simulink library "simCryogenics_lib"  (R2016a)
settings: Solver=VariableStepAuto  StartTime=0.0  StopTime=10.0  RelTol=1e-3
undefined symbols (not defined in the file or in its folder): gcbh, simscape
(part 4 of 4)

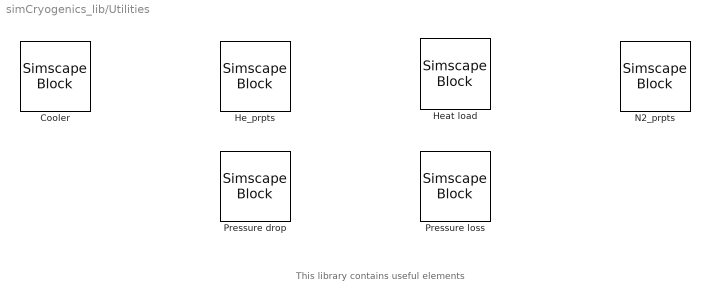
== system simCryogenics_lib/Utilities ==
  note: This library contains useful elements
  Cooler : SimscapeBlock  DialogController=NetworkEngine.DynNeDlgSource  LoadFcn=simscape.compiler.sli.internal.callback('LoadFcn',gcbh);  SourceFile=simCryogenics.Utilities.Cooler  mask(Cooler){ComponentPath=simCryogenics.Utilities.Cooler, ComponentVariants=simCryogenics.Utilities.Cooler, ComponentVariantNames=Cooler, ClassName=Cooler, SchemaVersion=1, Tout=300, Tout_unit=K, Tout_conf=compiletime}
      mask prompts: Tout "output temperature"
      mask help: This block is a cooler
      mask init:
      | simscape.compiler.sli.internal.preinitmask(gcb);
      settings: CopyFcn=simscape.compiler.sli.internal.callback('CopyFcn',gcbh);  DeleteFcn=simscape.compiler.sli.internal.callback('DeleteFcn',gcbh);  ModelCloseFcn=simscape.compiler.sli.internal.callback('ModelCloseFcn',gcbh);  PreSaveFcn=simscape.compiler.sli.internal.callback('PreSaveFcn',gcbh);  PostSaveFcn=simscape.compiler.sli.internal.callback('PostSaveFcn',gcbh);  PreCopyFcn=simscape.compiler.sli.internal.callback('PreCopyFcn',gcbh);  PreDeleteFcn=simscape.compiler.sli.internal.callback('PreDeleteFcn',gcbh);
      mask Help: web(nesl_help(gcbh))
      mask TypeOptions Tout_conf: compiletime | runtime
      mask Display:
      | disp('Simscape\n\n\n')
      | disp('\n\n\nCooler');
      | color('red');
      | port_label('RConn', 1,'out');
      | port_label('LConn', 1,'in');
  He_prpts : SimscapeBlock  DialogController=NetworkEngine.DynNeDlgSource  LoadFcn=simscape.compiler.sli.internal.callback('LoadFcn',gcbh);  SourceFile=simCryogenics.Utilities.He_prpts  mask(He_prpts){ComponentPath=simCryogenics.Utilities.He_prpts, ComponentVariants=simCryogenics.Utilities.He_prpts, ComponentVariantNames=He_prpts, ClassName=He_prpts, SchemaVersion=1, P_min=0.01, P_min_unit=bar, P_min_conf=compiletime, P_max=50, P_max_unit=bar, P_max_conf=compiletime, T_min=1, T_min_unit=K, T_min_conf=compiletime, T_max=100, T_max_unit=K, T_max_conf=compiletime, N=100, N_unit=1, N_conf=compiletime, Mol=4.0026 * (10 ^ (- 3)), Mol_unit=kg/mol, Mol_conf=compiletime}
      mask prompts: P_min "Min. pressure"; P_max "Max. pressure"; T_min "Min. temperature"; T_max "Max. temperature"; N "Grid size"; Mol "Molar mass"
      mask help:
      | The block controls fluidHelium domain properties for the attached circuit.
      |
      | You must have one of this block connectiong to your circuit
      |
      | For a good use of this component you must respect the following point :
      |
      | - All the parameters have to be greater than 0
      |
      | - Minimum parameters have to be lower than maximum parameters
      |
      | - If you use a very large scale (ie Min << Max), the precision of this component may decline
      mask init:
      | simscape.compiler.sli.internal.preinitmask(gcb);
      settings: CopyFcn=simscape.compiler.sli.internal.callback('CopyFcn',gcbh);  DeleteFcn=simscape.compiler.sli.internal.callback('DeleteFcn',gcbh);  ModelCloseFcn=simscape.compiler.sli.internal.callback('ModelCloseFcn',gcbh);  PreSaveFcn=simscape.compiler.sli.internal.callback('PreSaveFcn',gcbh);  PostSaveFcn=simscape.compiler.sli.internal.callback('PostSaveFcn',gcbh);  PreCopyFcn=simscape.compiler.sli.internal.callback('PreCopyFcn',gcbh);  PreDeleteFcn=simscape.compiler.sli.internal.callback('PreDeleteFcn',gcbh);
      mask Help: web(nesl_help(gcbh))
      mask TypeOptions P_min_conf: compiletime
      mask TypeOptions P_max_conf: compiletime
      mask TypeOptions T_min_conf: compiletime
      mask TypeOptions T_max_conf: compiletime
      mask TypeOptions N_conf: compiletime
      mask TypeOptions Mol_conf: compiletime
      mask Display:
      | color('red');
      | port_label('RConn', 1,'');
  Heat load : SimscapeBlock  DialogController=NetworkEngine.DynNeDlgSource  LoadFcn=simscape.compiler.sli.internal.callback('LoadFcn',gcbh);  SourceFile=simCryogenics.Utilities.HeatLoad  mask(Heat load){ComponentPath=simCryogenics.Utilities.HeatLoad, ComponentVariants=simCryogenics.Utilities.HeatLoad, ComponentVariantNames=HeatLoad, ClassName=HeatLoad, SchemaVersion=1}
      mask help:
      | For a good use of this component you must respect the following point :
      |
      | - Connect the in1 of the Thermal load block to a component that provied Temperature and pressure (not the mass flow)
      |
      | - Connect the out1 of the Thermal load block to a component that provied the mass flow (not the pressure neiter the temperature)
      mask init:
      | simscape.compiler.sli.internal.preinitmask(gcb);
      settings: CopyFcn=simscape.compiler.sli.internal.callback('CopyFcn',gcbh);  DeleteFcn=simscape.compiler.sli.internal.callback('DeleteFcn',gcbh);  ModelCloseFcn=simscape.compiler.sli.internal.callback('ModelCloseFcn',gcbh);  PreSaveFcn=simscape.compiler.sli.internal.callback('PreSaveFcn',gcbh);  PostSaveFcn=simscape.compiler.sli.internal.callback('PostSaveFcn',gcbh);  PreCopyFcn=simscape.compiler.sli.internal.callback('PreCopyFcn',gcbh);  PreDeleteFcn=simscape.compiler.sli.internal.callback('PreDeleteFcn',gcbh);
      mask Help: web(nesl_help(gcbh))
      mask Display:
      | color('red');
      | port_label('LConn', 2,'Win');
      | port_label('RConn', 1,'out1');
      | port_label('LConn', 1,'in1');
  N2_prpts : SimscapeBlock  DialogController=NetworkEngine.DynNeDlgSource  LoadFcn=simscape.compiler.sli.internal.callback('LoadFcn',gcbh);  SourceFile=simCryogenics.Utilities.N2_prpts  mask(N2_prpts){ComponentPath=simCryogenics.Utilities.N2_prpts, ComponentVariants=simCryogenics.Utilities.N2_prpts, ComponentVariantNames=N2_prpts, ClassName=N2_prpts, SchemaVersion=1, P_min=0.5, P_min_unit=bar, P_min_conf=compiletime, T_min=70, T_min_unit=K, T_min_conf=compiletime, T_max=320, T_max_unit=K, T_max_conf=compiletime, P_max=20, P_max_unit=bar, P_max_conf=compiletime, Mol=4.0026 * (10 ^ (- 3)), Mol_unit=kg/mol, Mol_conf=compiletime}
      mask prompts: P_min "Minimum allowable pressure"; T_min "Minimum allowable temperature"; T_max "Maximum allowable temperature"; P_max "Maximum allowable pressure"; Mol "Molar mass of the fluid (here helium)"
      mask help:
      | The block controls fluidHelium domain properties for the attached circuit.
      |
      | You must have one of this block connectiong to your circuit
      |
      | For a good use of this component you must respect the following point :
      |
      | - All the parameters have to be greater than 0
      |
      | - Minimum parameters have to be lower than maximum parameters
      |
      | - If you use a very large scale (ie Min << Max), the precision of this component may decline
      mask init:
      | simscape.compiler.sli.internal.preinitmask(gcb);
      settings: CopyFcn=simscape.compiler.sli.internal.callback('CopyFcn',gcbh);  DeleteFcn=simscape.compiler.sli.internal.callback('DeleteFcn',gcbh);  ModelCloseFcn=simscape.compiler.sli.internal.callback('ModelCloseFcn',gcbh);  PreSaveFcn=simscape.compiler.sli.internal.callback('PreSaveFcn',gcbh);  PostSaveFcn=simscape.compiler.sli.internal.callback('PostSaveFcn',gcbh);  PreCopyFcn=simscape.compiler.sli.internal.callback('PreCopyFcn',gcbh);  PreDeleteFcn=simscape.compiler.sli.internal.callback('PreDeleteFcn',gcbh);
      mask Help: web(nesl_help(gcbh))
      mask TypeOptions P_min_conf: compiletime
      mask TypeOptions T_min_conf: compiletime
      mask TypeOptions T_max_conf: compiletime
      mask TypeOptions P_max_conf: compiletime
      mask TypeOptions Mol_conf: compiletime
      mask Display:
      | color('red');
      | port_label('RConn', 1,'');
  Pressure drop : SimscapeBlock  DialogController=NetworkEngine.DynNeDlgSource  LoadFcn=simscape.compiler.sli.internal.callback('LoadFcn',gcbh);  SourceFile=simCryogenics.Utilities.PressureDrop  mask(Pressure drop){ComponentPath=simCryogenics.Utilities.PressureDrop, ComponentVariants=simCryogenics.Utilities.PressureDrop, ComponentVariantNames=PressureDrop, ClassName=PressureDrop, SchemaVersion=1, K=1, K_unit=s*bar/kg, K_conf=compiletime}
      mask prompts: K "Loss coefficient"
      mask help:
      | For a good use of this component you must respect the following point :
      |
      | - Connect the in1 of the PressureDrop block to a component that provied Temperature and pressure (not the mass flow)
      |
      | - Connect the out1 of the PressureDrop block to a component that provied the Pressure (not the mass flow neiter the temperature)
      mask init:
      | simscape.compiler.sli.internal.preinitmask(gcb);
      settings: CopyFcn=simscape.compiler.sli.internal.callback('CopyFcn',gcbh);  DeleteFcn=simscape.compiler.sli.internal.callback('DeleteFcn',gcbh);  ModelCloseFcn=simscape.compiler.sli.internal.callback('ModelCloseFcn',gcbh);  PreSaveFcn=simscape.compiler.sli.internal.callback('PreSaveFcn',gcbh);  PostSaveFcn=simscape.compiler.sli.internal.callback('PostSaveFcn',gcbh);  PreCopyFcn=simscape.compiler.sli.internal.callback('PreCopyFcn',gcbh);  PreDeleteFcn=simscape.compiler.sli.internal.callback('PreDeleteFcn',gcbh);
      mask Help: web(nesl_help(gcbh))
      mask TypeOptions K_conf: compiletime | runtime
      mask Display:
      | color('red');
      | port_label('RConn', 1,'out1');
      | port_label('LConn', 1,'in1');
  Pressure loss : SimscapeBlock  DialogController=NetworkEngine.DynNeDlgSource  LoadFcn=simscape.compiler.sli.internal.callback('LoadFcn',gcbh);  SourceFile=simCryogenics.Utilities.PressureLoss  mask(Pressure loss){ComponentPath=simCryogenics.Utilities.PressureLoss, ComponentVariants=simCryogenics.Utilities.PressureLoss, ComponentVariantNames=PressureLoss, ClassName=PressureLoss, SchemaVersion=1, K=1, K_unit=s*bar/kg, K_conf=compiletime}
      mask prompts: K "Loss coefficient"
      mask init:
      | simscape.compiler.sli.internal.preinitmask(gcb);
      settings: CopyFcn=simscape.compiler.sli.internal.callback('CopyFcn',gcbh);  DeleteFcn=simscape.compiler.sli.internal.callback('DeleteFcn',gcbh);  ModelCloseFcn=simscape.compiler.sli.internal.callback('ModelCloseFcn',gcbh);  PreSaveFcn=simscape.compiler.sli.internal.callback('PreSaveFcn',gcbh);  PostSaveFcn=simscape.compiler.sli.internal.callback('PostSaveFcn',gcbh);  PreCopyFcn=simscape.compiler.sli.internal.callback('PreCopyFcn',gcbh);  PreDeleteFcn=simscape.compiler.sli.internal.callback('PreDeleteFcn',gcbh);
      mask Help: web(nesl_help(gcbh))
      mask TypeOptions K_conf: compiletime | runtime
      mask Display:
      | disp('Simscape\n\n\n')
      | disp('\n\n\nPressureLoss');
      | color('red');
      | port_label('RConn', 1,'out1');
      | port_label('LConn', 1,'in1');
